simulink model "ex_40"  (R2018b)
settings: Solver=VariableStepAuto  StartTime=0.0  StopTime=10.0  RelTol=1e-3
settings Model: Creator=lenovo  LastModifiedBy=QJ-
settings DebuggingCC: LibraryContextMissingDiagnostic=none
settings SFSimCC: SimUseLocalCustomCode=off
settings RTWCC: RTWUseLocalCustomCode=off

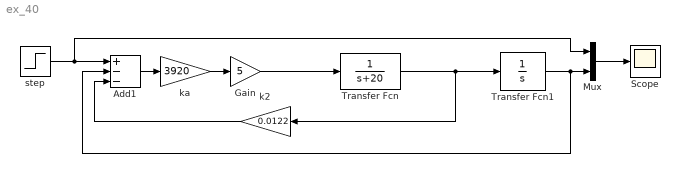
== system ex_40 ==
  Add1 : Sum  Inputs=+--
  Gain : Gain  Gain=5
  Mux : Mux  Inputs=2
  Scope : Scope
  Transfer Fcn : TransferFcn  Denominator=[1 20]
  Transfer Fcn1 : TransferFcn  Denominator=[1 0]
  k2 : Gain  Gain=0.0122
  ka : Gain  Gain=3920
  step : Step  SampleTime=1  mask(DiscretizedSource){}
      mask init:
      | %zoh
  wires:
  Mux/1 -> Scope/1
  Add1/1 -> ka/1
  k2/1 -> Add1/3
  ka/1 -> Gain/1
  Transfer Fcn/1 -> Transfer Fcn1/1, k2/1
  Gain/1 -> Transfer Fcn/1
  step/1 -> Mux/1, Add1/1
  Transfer Fcn1/1 -> Mux/2, Add1/2
